simulink model "mvdc_path_feedback"  (R2018b)
settings: configuration reference "Active" (kept outside this file)
undefined symbols (not defined in the file): l_front_m, l_rear_m, P_VDC_ActivateBarriersCorrection_b, P_VDC_ActivateBetaCompensation, P_VDC_ActivateKappaDynamicFF_b, P_VDC_ActivateKappaFFFIR, P_VDC_ActivateKappaFFPT1, P_VDC_BarrierCorrectionGain_radpmpm, P_VDC_BarrierEmergency_radpm, P_VDC_BarriersCorrectionPT1_s, P_VDC_ControlMaxSpeed_mps, P_VDC_ControlMinSpeed_mps, P_VDC_CorrectionBarrierDistance_m, P_VDC_KappaFFPathFeedback_Ts, P_VDC_KappaT1_s, P_VDC_LatConvergence, P_VDC_LatDamping, P_VDC_LatKappaMaxFB_radpm, P_VDC_LatKappaMinFB_radpm, P_VDC_LongFF_PT1_s, P_VDC_MinBarrierDistance_m, P_VDC_MinSpeedGainCorrection_mps, P_VDC_NumDerivativeTFilter_s, P_VDC_UseBetaFeedback, P_VDC_UseExternalControllerParam, P_VDC_UseLongFF_PT1_b, P_VDC_UseNumDerivativePathFeedback_b, P_VDC_UseSSCDynamicsComp_b, P_VDC_UseWatchdogExternalControlParam, tS, TUMHealthStatus
libraries: simulink x10, rr_general x2
settings Model: DataDictionary=mvdc_path_feedback.sldd  Creator=wischnewski  LastModifiedBy=ge34qer

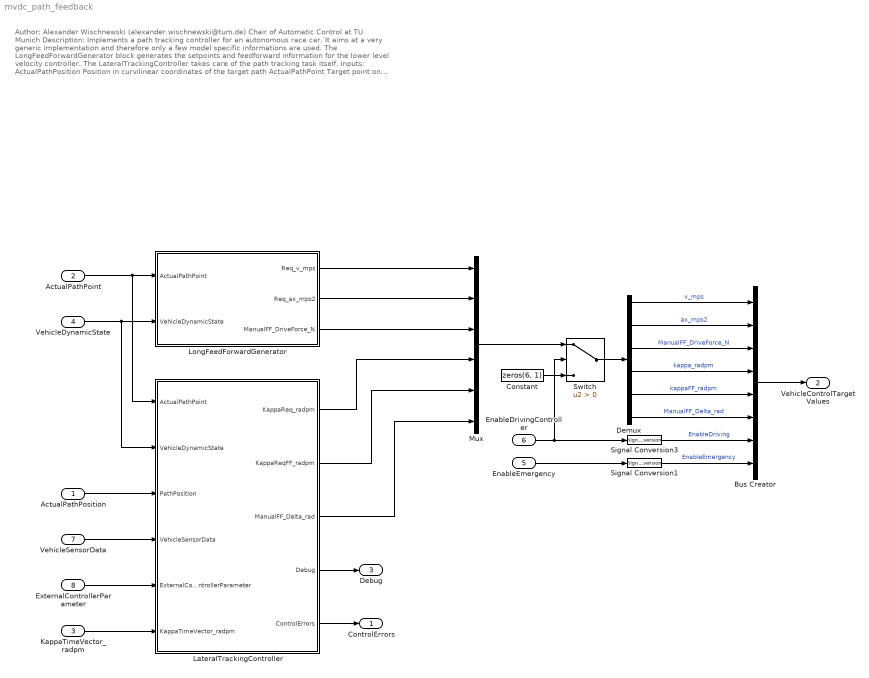
== system mvdc_path_feedback ==
  note: Author: Alexander Wischnewski (alexander.wischnewski@tum.de)
      | Chair of Automatic Control at TU Munich
      |
      | Description: Implements a path tracking controller for an autonomous race car. It aims at a very generic implementation
      | and therefore only a few model specific informations are used.
      |
      | The LongFeedForwardGenerator block generates the setpoints and feedforward information for the
      | lower level velocity controller.
      |
      | The LateralTrackingController takes care of the path tracking task itself.
      |
      | Inputs:
      | ActualPathPosition Position in curvilinear coordinates of the target path
      | ActualPathPoint Target point on the target path (found by path matching)
      | VehicleDynamicState Fused state vector of the vehicle (including position, velocity, acceleration, etc.)
      | EnableDrivingController Enable bit for controller operation
      | EnableEmergency Enable bit for emergecy control mode
      | VehicleSensorData All raw sensor data available
      | ExternalControllerParameter Interface for external modification of controller parameters (used for controller learning)
      | KappaTimeVector_radpm Vector with curvature values for a time windows of +-0.5sec
      |
      | Outputs:
      | VehicleControlTargetValues Low level controller interface of the vehicle
      | ControlErrors Outputs relevant information for controller learning
  ActualPathPosition : Inport  OutDataTypeStr=Bus: PathPos  PortDimensions=1  BusOutputAsStruct=on
  ActualPathPoint : Inport  Port=2  OutDataTypeStr=Bus: PathPoint  PortDimensions=1  BusOutputAsStruct=on
  KappaTimeVector_radpm : Inport  Port=3  PortDimensions=501  BusOutputAsStruct=on
  VehicleDynamicState : Inport  Port=4  OutDataTypeStr=Bus: VehicleDynamicState
  EnableEmergency : Inport  Port=5  OutDataTypeStr=boolean  PortDimensions=1  BusOutputAsStruct=on
  EnableDrivingController : Inport  Port=6  OutDataTypeStr=boolean  PortDimensions=1  BusOutputAsStruct=on
  VehicleSensorData : Inport  Port=7  OutDataTypeStr=Bus: VehicleSensorData  PortDimensions=1  BusOutputAsStruct=on
  ExternalControllerParameter : Inport  Port=8  OutDataTypeStr=Bus: ControllerParameter  BusOutputAsStruct=on
  Bus Creator : BusCreator  Inputs=8  OutDataTypeStr=Bus: TargetValuesVehicleDynamics
      settings: InheritFromInputs=off
  Constant : Constant  Value=zeros(6, 1)
  Demux : Demux  Outputs=6
  LateralTrackingController : Subsystem
  LongFeedForwardGenerator : Subsystem
  Mux : Mux  Inputs=6
  Signal Conversion1 : SignalConversion  OverrideOpt=off
  Signal Conversion3 : SignalConversion  OverrideOpt=off
  Switch : Switch  Criteria=u2 > Threshold
  ControlErrors : Outport  OutDataTypeStr=Bus: ControlErrors
  VehicleControlTargetValues : Outport  Port=2  OutDataTypeStr=Bus: TargetValuesVehicleDynamics
  Debug : Outport  Port=3  OutDataTypeStr=Bus: mvdc_path_feedback_debug
  wires:
  ActualPathPoint/1 -> LateralTrackingController/1(ActualPathPoint), LongFeedForwardGenerator/1(ActualPathPoint)
  ActualPathPosition/1 -> LateralTrackingController/3(PathPosition)
  VehicleDynamicState/1 -> LateralTrackingController/2(VehicleDynamicState), LongFeedForwardGenerator/2(VehicleDynamicState)
  Bus Creator/1 -> VehicleControlTargetValues/1
  Demux/5 -> Bus Creator/5  "kappaFF_radpm"
  Demux/4 -> Bus Creator/4  "kappa_radpm"
  Demux/1 -> Bus Creator/1  "v_mps"
  Demux/2 -> Bus Creator/2  "ax_mps2"
  EnableDrivingController/1 -> Switch/2, Signal Conversion3/1
  Signal Conversion3/1 -> Bus Creator/7  "EnableDriving"
  Signal Conversion1/1 -> Bus Creator/8  "EnableEmergency"
  EnableEmergency/1 -> Signal Conversion1/1
  LongFeedForwardGenerator/1(Req_v_mps) -> Mux/1
  LongFeedForwardGenerator/2(Req_ax_mps2) -> Mux/2
  LateralTrackingController/1(KappaReq_radpm) -> Mux/4
  LateralTrackingController/2(KappaReqFF_radpm) -> Mux/5
  Mux/1 -> Switch/1
  Constant/1 -> Switch/3
  Switch/1 -> Demux/1
  LateralTrackingController/4(Debug) -> Debug/1
  VehicleSensorData/1 -> LateralTrackingController/4(VehicleSensorData)
  Demux/6 -> Bus Creator/6  "ManualFF_Delta_rad"
  Demux/3 -> Bus Creator/3  "ManualFF_DriveForce_N"
  ExternalControllerParameter/1 -> LateralTrackingController/5(ExternalControllerParameter)
  KappaTimeVector_radpm/1 -> LateralTrackingController/6(KappaTimeVector_radpm)
  LongFeedForwardGenerator/3(ManualFF_DriveForce_N) -> Mux/3
  LateralTrackingController/3(ManualFF_Delta_rad) -> Mux/6
  LateralTrackingController/5(ControlErrors) -> ControlErrors/1

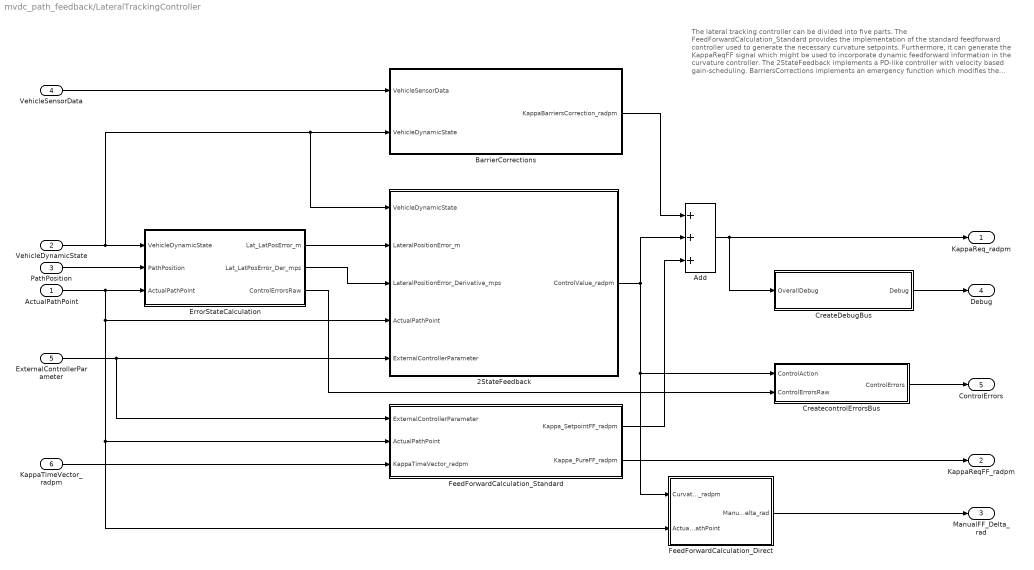
== system mvdc_path_feedback/LateralTrackingController ==
  note: The lateral tracking controller can be divided into five parts.
      |
      | The FeedForwardCalculation_Standard provides the implementation
      | of the standard feedforward controller used to generate the necessary curvature setpoints.
      | Furthermore, it can generate the KappaReqFF signal which might be used to incorporate
      | dynamic feedforward information in the curvature controller.
      |
      | The 2StateFeedback implements a PD-like controller with velocity based gain-scheduling.
      |
      | BarriersCorrections implements an emergency function which modifies the target curvature
      | signals in case barriers are near.
      |
      | ErrorStateCalculation generates the necessary control error values and its derivatives.
      |
      | Finally, FeedForwardCalculation_Direct uses a potentially available steering feedforward
      | value instead of the path curvature to generate the feedforward information. This is handed
      | directly to the lower level controller.
  ActualPathPoint : Inport  OutDataTypeStr=Bus: PathPoint
  VehicleDynamicState : Inport  Port=2  OutDataTypeStr=Bus: VehicleDynamicState
  PathPosition : Inport  Port=3
  VehicleSensorData : Inport  Port=4  OutDataTypeStr=Bus: VehicleSensorData
  ExternalControllerParameter : Inport  Port=5  BusOutputAsStruct=on
  KappaTimeVector_radpm : Inport  Port=6  PortDimensions=501  BusOutputAsStruct=on
  2StateFeedback : Subsystem
  Add : Sum  Inputs=3
  BarrierCorrections : Subsystem
  CreateDebugBus : Subsystem
  CreatecontrolErrorsBus : Subsystem
  ErrorStateCalculation : Subsystem
  FeedForwardCalculation_Direct : Subsystem
  FeedForwardCalculation_Standard : Subsystem
  KappaReq_radpm : Outport
  KappaReqFF_radpm : Outport  Port=2
  ManualFF_Delta_rad : Outport  Port=3
  Debug : Outport  Port=4
  ControlErrors : Outport  Port=5
  wires:
  Add/1 -> KappaReq_radpm/1, CreateDebugBus/1(OverallDebug)
  2StateFeedback/1(ControlValue_radpm) -> FeedForwardCalculation_Direct/1(CurvatureFeedback_radpm), CreatecontrolErrorsBus/1(ControlAction), Add/2
  FeedForwardCalculation_Standard/2(Kappa_PureFF_radpm) -> KappaReqFF_radpm/1
  VehicleDynamicState/1 -> BarrierCorrections/2(VehicleDynamicState), 2StateFeedback/1(VehicleDynamicState), ErrorStateCalculation/1(VehicleDynamicState)
  BarrierCorrections/1(KappaBarriersCorrection_radpm) -> Add/1
  ExternalControllerParameter/1 -> 2StateFeedback/5(ExternalControllerParameter), FeedForwardCalculation_Standard/1(ExternalControllerParameter)
  VehicleSensorData/1 -> BarrierCorrections/1(VehicleSensorData)
  ErrorStateCalculation/1(Lat_LatPosError_m) -> 2StateFeedback/2(LateralPositionError_m)
  PathPosition/1 -> ErrorStateCalculation/2(PathPosition)
  ErrorStateCalculation/2(Lat_LatPosError_Der_mps) -> 2StateFeedback/3(LateralPositionError_Derivative_mps)
  ActualPathPoint/1 -> FeedForwardCalculation_Direct/2(ActualPathPoint), FeedForwardCalculation_Standard/2(ActualPathPoint), 2StateFeedback/4(ActualPathPoint), ErrorStateCalculation/3(ActualPathPoint)
  FeedForwardCalculation_Standard/1(Kappa_SetpointFF_radpm) -> Add/3
  KappaTimeVector_radpm/1 -> FeedForwardCalculation_Standard/3(KappaTimeVector_radpm)
  CreateDebugBus/1(Debug) -> Debug/1
  FeedForwardCalculation_Direct/1(ManualFF_Delta_rad) -> ManualFF_Delta_rad/1
  ErrorStateCalculation/3(ControlErrorsRaw) -> CreatecontrolErrorsBus/2(ControlErrorsRaw)
  CreatecontrolErrorsBus/1(ControlErrors) -> ControlErrors/1

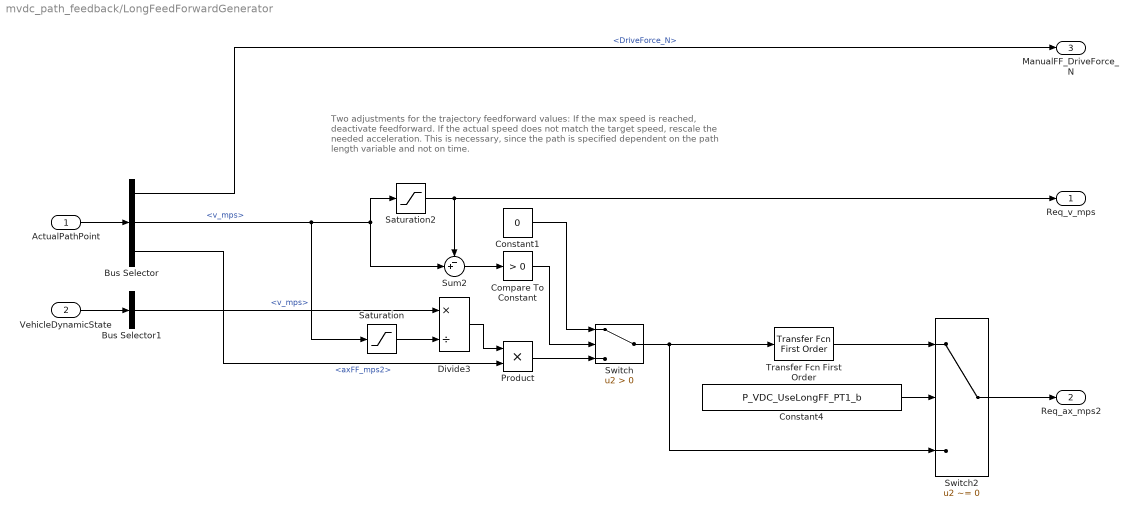
== system mvdc_path_feedback/LongFeedForwardGenerator ==
  note: Two adjustments for the trajectory feedforward values:
      | If the max speed is reached, deactivate feedforward.
      | If the actual speed does not match the target speed, rescale the needed acceleration.
      | This is necessary, since the path is specified dependent on the path length variable and
      | not on time.
  ActualPathPoint : Inport
  VehicleDynamicState : Inport  Port=2
  Bus Selector : BusSelector  OutputSignals=DriveForce_N,v_mps,axFF_mps2
  Bus Selector1 : BusSelector  OutputSignals=v_mps
  Compare To Constant : simulink/Logic and Bit Operations/Compare To Constant  relop=>  const=0  OutDataTypeStr=boolean
  Constant1 : Constant  Value=0
  Constant4 : Constant  Value=P_VDC_UseLongFF_PT1_b
  Divide3 : Product  Inputs=*/
  Product : Product
  Saturation : Saturate  UpperLimit=inf  LowerLimit=2
  Saturation2 : Saturate  UpperLimit=P_VDC_ControlMaxSpeed_mps  LowerLimit=P_VDC_ControlMinSpeed_mps
  Sum2 : Sum  Inputs=-+|
  Switch : Switch  Criteria=u2 > Threshold
  Switch2 : Switch  Criteria=u2 ~= 0
  Transfer Fcn First Order : simulink/Discrete/Transfer Fcn First Order  PoleZ=exp(-tS/P_VDC_LongFF_PT1_s)  ICPrevOutput=0.0  DoSatur=off
      settings: SourceProductName=Simulink
  Req_v_mps : Outport
  Req_ax_mps2 : Outport  Port=2
  ManualFF_DriveForce_N : Outport  Port=3
  wires:
  Constant1/1 -> Switch/1
  Sum2/1 -> Compare To Constant/1
  Compare To Constant/1 -> Switch/2
  Product/1 -> Switch/3
  Saturation/1 -> Divide3/2
  Divide3/1 -> Product/1
  Bus Selector/3 -> Product/2  "<axFF_mps2>"
  Bus Selector/2 -> Saturation/1, Saturation2/1, Sum2/2  "<v_mps>"
  Saturation2/1 -> Req_v_mps/1, Sum2/1
  Switch/1 -> Switch2/3, Transfer Fcn First Order/1
  Constant4/1 -> Switch2/2
  Transfer Fcn First Order/1 -> Switch2/1
  Switch2/1 -> Req_ax_mps2/1
  ActualPathPoint/1 -> Bus Selector/1
  VehicleDynamicState/1 -> Bus Selector1/1
  Bus Selector1/1 -> Divide3/1  "<v_mps>"
  Bus Selector/1 -> ManualFF_DriveForce_N/1  "<DriveForce_N>"

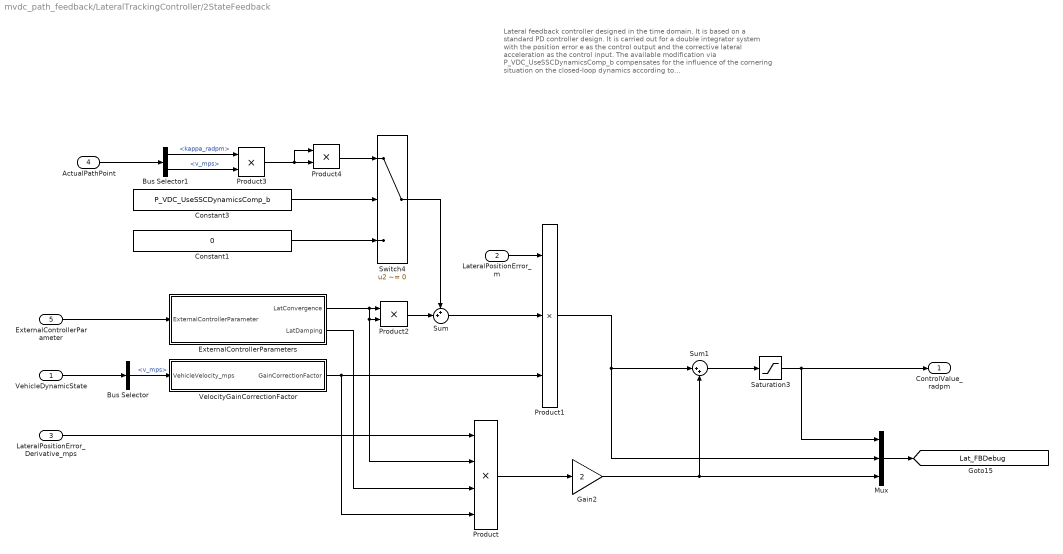
== system mvdc_path_feedback/LateralTrackingController/2StateFeedback ==
  note: Lateral feedback controller designed in the time domain. It is based on a standard PD controller design. It is carried out for a double integrator system with the position error e as the control output and the corrective lateral acceleration as the control input. The available modification via P_VDC_UseSSCDynamicsComp_b compensates for the influence of the cornering situation on the closed-loop dynamics according to
      | https://ieeexplore.ieee.org/document/6580852
      |
      | The final value is transformed to an equivalent curvature signal by using the velocity gain correction factor .
      |
      | The external controller parameters block allows to interface the controller from an other algorithm. This is used for controller learning.
  VehicleDynamicState : Inport
  LateralPositionError_m : Inport  Port=2
  LateralPositionError_Derivative_mps : Inport  Port=3
  ActualPathPoint : Inport  Port=4  OutDataTypeStr=Bus: PathPoint
  ExternalControllerParameter : Inport  Port=5  BusOutputAsStruct=on
  Bus Selector : BusSelector  OutputSignals=v_mps
  Bus Selector1 : BusSelector  OutputSignals=kappa_radpm,v_mps
  Constant1 : Constant  Value=0
  Constant3 : Constant  Value=P_VDC_UseSSCDynamicsComp_b
  ExternalControllerParameters : Subsystem
  Gain2 : Gain  Gain=2
  Mux : Mux  Inputs=3
  Product : Product  Inputs=4
  Product1 : Product  Inputs=3
  Product2 : Product
  Product3 : Product
  Product4 : Product
  Saturation3 : Saturate  UpperLimit=P_VDC_LatKappaMaxFB_radpm  LowerLimit=P_VDC_LatKappaMinFB_radpm
  Sum : Sum  Inputs=++|
  Sum1 : Sum  Inputs=|++
  Switch4 : Switch  Criteria=u2 ~= 0
  VelocityGainCorrectionFactor : Subsystem
  ControlValue_radpm : Outport
  tag scope: Lat_FBDebug=global
  wires:
  LateralPositionError_m/1 -> Product1/1
  Product/1 -> Gain2/1
  ExternalControllerParameters/2(LatDamping) -> Product/3
  ExternalControllerParameters/1(LatConvergence) -> Product2/2, Product/2, Product2/1
  VelocityGainCorrectionFactor/1(GainCorrectionFactor) -> Product1/3, Product/4
  Sum1/1 -> Saturation3/1
  ExternalControllerParameter/1 -> ExternalControllerParameters/1(ExternalControllerParameter)
  VehicleDynamicState/1 -> Bus Selector/1
  Bus Selector/1 -> VelocityGainCorrectionFactor/1(VehicleVelocity_mps)  "<v_mps>"
  Saturation3/1 -> Mux/1, ControlValue_radpm/1
  Product1/1 -> Mux/2, Sum1/1
  Gain2/1 -> Mux/3, Sum1/2
  Mux/1 -> [Lat_FBDebug]
  Product2/1 -> Sum/2
  Sum/1 -> Product1/2
  Product3/1 -> Product4/1, Product4/2
  ActualPathPoint/1 -> Bus Selector1/1
  Bus Selector1/1 -> Product3/1  "<kappa_radpm>"
  Bus Selector1/2 -> Product3/2  "<v_mps>"
  Constant3/1 -> Switch4/2
  Product4/1 -> Switch4/1
  Switch4/1 -> Sum/1
  Constant1/1 -> Switch4/3
  LateralPositionError_Derivative_mps/1 -> Product/1

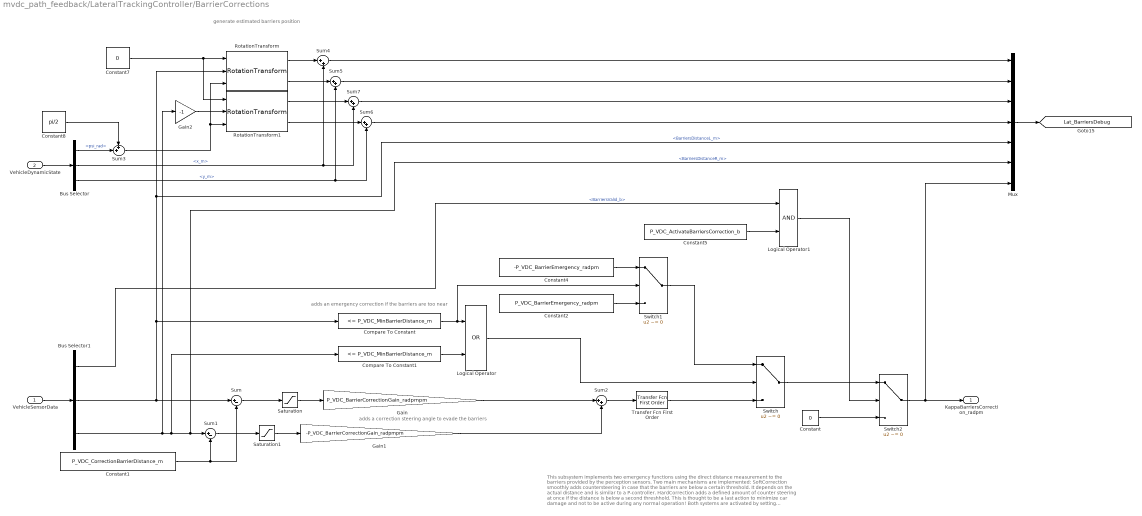
== system mvdc_path_feedback/LateralTrackingController/BarrierCorrections ==
  note: This subsystem implements two emergency functions using the direct distance measurement
      | to the barriers provided by the perception sensors.
      |
      | Two main mechanisms are implemented:
      | SoftCorrection smoothly adds countersteering in case that the barriers are below a certain threshold. It depends
      | on the actual distance and is similar to a P-controller.
      | HardCorrection adds a defined amount of counter steering at once if the distance is below a second threshhold.
      | This is thought to be a last action to minimize car damage and not to be active during any normal operation!
      |
      | Both systems are activated by setting P_VDC_ActivateBarriersCorrection_b to true.
  note: generate estimated barriers position
  note: adds an emergency correction if the barriers are too near
  note: adds a correction steering angle to evade the barriers
  VehicleSensorData : Inport
  VehicleDynamicState : Inport  Port=2
  Bus Selector : BusSelector  OutputSignals=Pos.psi_rad,Pos.x_m,Pos.y_m
  Bus Selector1 : BusSelector  OutputSignals=BarriersValid_b,BarriersDistanceL_m,BarriersDistanceR_m
  Compare To Constant : simulink/Logic and Bit Operations/Compare To Constant  relop=<=  const=P_VDC_MinBarrierDistance_m  OutDataTypeStr=boolean
  Compare To Constant1 : simulink/Logic and Bit Operations/Compare To Constant  relop=<=  const=P_VDC_MinBarrierDistance_m  OutDataTypeStr=boolean
  Constant : Constant  Value=0
  Constant1 : Constant  Value=P_VDC_CorrectionBarrierDistance_m
  Constant2 : Constant  Value=P_VDC_BarrierEmergency_radpm
  Constant4 : Constant  Value=-P_VDC_BarrierEmergency_radpm
  Constant5 : Constant  Value=P_VDC_ActivateBarriersCorrection_b
  Constant7 : Constant  Value=0
  Constant8 : Constant  Value=pi/2
  Gain : Gain  Gain=P_VDC_BarrierCorrectionGain_radpmpm
  Gain1 : Gain  Gain=-P_VDC_BarrierCorrectionGain_radpmpm
  Gain2 : Gain  Gain=-1
  Logical Operator : Logic  Operator=OR  AllPortsSameDT=off  OutDataTypeStr=boolean
  Logical Operator1 : Logic  AllPortsSameDT=off  OutDataTypeStr=boolean
  Mux : Mux  Inputs=7
  RotationTransform : rr_general/RotationTransform  SystemSampleTime=-1
  RotationTransform1 : rr_general/RotationTransform  SystemSampleTime=-1
  Saturation : Saturate  UpperLimit=0  LowerLimit=-(P_VDC_CorrectionBarrierDistance_m-P_VDC_MinBarrierDistance_m)
  Saturation1 : Saturate  UpperLimit=0  LowerLimit=-(P_VDC_CorrectionBarrierDistance_m-P_VDC_MinBarrierDistance_m)
  Sum : Sum  Inputs=|+-
  Sum1 : Sum  Inputs=|+-
  Sum{2,4..7} (5 alike) : Sum  Inputs=|++
  Sum3 : Sum  Inputs=++|
  Switch : Switch  Criteria=u2 ~= 0
  Switch1 : Switch  Criteria=u2 ~= 0
  Switch2 : Switch  Criteria=u2 ~= 0
  Transfer Fcn First Order : simulink/Discrete/Transfer Fcn First Order  PoleZ=exp(-tS/P_VDC_BarriersCorrectionPT1_s)  ICPrevOutput=0.0  DoSatur=off
      settings: SourceProductName=Simulink
  KappaBarriersCorrection_radpm : Outport
  tag scope: Lat_BarriersDebug=global
  wires:
  Bus Selector1/3 -> Gain2/1, Compare To Constant1/1, Mux/6, Sum1/1  "<BarriersDistanceR_m>"
  Constant1/1 -> Sum/2, Sum1/2
  Sum/1 -> Saturation/1
  Sum1/1 -> Saturation1/1
  Saturation/1 -> Gain/1
  Saturation1/1 -> Gain1/1
  Gain/1 -> Sum2/1
  Gain1/1 -> Sum2/2
  Sum2/1 -> Transfer Fcn First Order/1
  Compare To Constant1/1 -> Logical Operator/2
  Compare To Constant/1 -> Switch1/2, Logical Operator/1
  Transfer Fcn First Order/1 -> Switch/3
  Logical Operator/1 -> Switch/2
  Switch1/1 -> Switch/1
  Constant2/1 -> Switch1/3
  Constant4/1 -> Switch1/1
  Switch/1 -> Switch2/1
  Switch2/1 -> Mux/7, KappaBarriersCorrection_radpm/1
  Constant/1 -> Switch2/3
  Logical Operator1/1 -> Switch2/2
  Gain2/1 -> RotationTransform1/2
  Constant7/1 -> RotationTransform1/1, RotationTransform/1
  VehicleDynamicState/1 -> Bus Selector/1
  Sum3/1 -> RotationTransform/3, RotationTransform1/3
  Bus Selector/1 -> Sum3/2  "<psi_rad>"
  Constant8/1 -> Sum3/1
  RotationTransform/1 -> Sum4/1
  Bus Selector/2 -> Sum7/2, Sum4/2  "<x_m>"
  RotationTransform/2 -> Sum5/1
  Bus Selector/3 -> Sum6/2, Sum5/2  "<y_m>"
  RotationTransform1/2 -> Sum6/1
  RotationTransform1/1 -> Sum7/1
  Sum6/1 -> Mux/4
  Sum7/1 -> Mux/3
  Sum5/1 -> Mux/2
  Sum4/1 -> Mux/1
  Bus Selector1/2 -> Mux/5, RotationTransform/2, Compare To Constant/1, Sum/1  "<BarriersDistanceL_m>"
  Constant5/1 -> Logical Operator1/2
  Bus Selector1/1 -> Logical Operator1/1  "<BarriersValid_b>"
  VehicleSensorData/1 -> Bus Selector1/1
  Mux/1 -> [Lat_BarriersDebug]

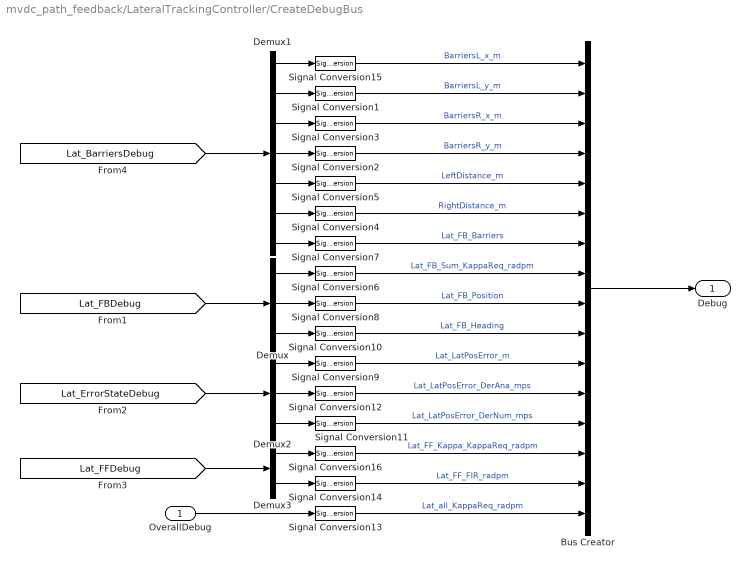
== system mvdc_path_feedback/LateralTrackingController/CreateDebugBus ==
  OverallDebug : Inport
  Bus Creator : BusCreator  Inputs=16
  Demux : Demux  Outputs=3
  Demux1 : Demux  Outputs=7
  Demux2 : Demux  Outputs=3
  Demux3 : Demux  Outputs=2
  Signal Conversion{1..16} (16 alike) : SignalConversion  OverrideOpt=off
  Debug : Outport
  wires:
  [Lat_FBDebug] -> Demux/1
  Demux3/2 -> Signal Conversion14/1
  Demux2/1 -> Signal Conversion9/1
  Demux1/3 -> Signal Conversion3/1
  Demux1/7 -> Signal Conversion7/1
  OverallDebug/1 -> Signal Conversion13/1
  Demux1/2 -> Signal Conversion1/1
  Demux1/1 -> Signal Conversion15/1
  Demux/2 -> Signal Conversion8/1
  Demux2/2 -> Signal Conversion12/1
  Demux2/3 -> Signal Conversion11/1
  Demux3/1 -> Signal Conversion16/1
  Demux1/6 -> Signal Conversion4/1
  [Lat_FFDebug] -> Demux3/1
  Bus Creator/1 -> Debug/1
  Demux1/4 -> Signal Conversion2/1
  Demux1/5 -> Signal Conversion5/1
  Demux/1 -> Signal Conversion6/1
  Demux/3 -> Signal Conversion10/1
  [Lat_ErrorStateDebug] -> Demux2/1
  [Lat_BarriersDebug] -> Demux1/1
  Signal Conversion15/1 -> Bus Creator/1  "BarriersL_x_m"
  Signal Conversion1/1 -> Bus Creator/2  "BarriersL_y_m"
  Signal Conversion2/1 -> Bus Creator/4  "BarriersR_y_m"
  Signal Conversion3/1 -> Bus Creator/3  "BarriersR_x_m"
  Signal Conversion4/1 -> Bus Creator/6  "RightDistance_m"
  Signal Conversion7/1 -> Bus Creator/7  "Lat_FB_Barriers"
  Signal Conversion5/1 -> Bus Creator/5  "LeftDistance_m"
  Signal Conversion6/1 -> Bus Creator/8  "Lat_FB_Sum_KappaReq_radpm"
  Signal Conversion8/1 -> Bus Creator/9  "Lat_FB_Position"
  Signal Conversion11/1 -> Bus Creator/13  "Lat_LatPosError_DerNum_mps"
  Signal Conversion9/1 -> Bus Creator/11  "Lat_LatPosError_m"
  Signal Conversion10/1 -> Bus Creator/10  "Lat_FB_Heading"
  Signal Conversion12/1 -> Bus Creator/12  "Lat_LatPosError_DerAna_mps"
  Signal Conversion13/1 -> Bus Creator/16  "Lat_all_KappaReq_radpm"
  Signal Conversion14/1 -> Bus Creator/15  "Lat_FF_FIR_radpm"
  Signal Conversion16/1 -> Bus Creator/14  "Lat_FF_Kappa_KappaReq_radpm"

== system mvdc_path_feedback/LateralTrackingController/CreatecontrolErrorsBus ==
  ControlAction : Inport
  ControlErrorsRaw : Inport  Port=2
  Bus Creator : BusCreator  Inputs=4
  Demux : Demux  Outputs=3
  ControlErrors : Outport
  wires:
  Bus Creator/1 -> ControlErrors/1
  Demux/1 -> Bus Creator/1  "e_LateralDeviation_m"
  Demux/2 -> Bus Creator/2  "de_LateralDeviationDer_mps"
  Demux/3 -> Bus Creator/3  "ePsi_HeadingDeviation_rad"
  ControlErrorsRaw/1 -> Demux/1
  ControlAction/1 -> Bus Creator/4  "u_ControlInput_radpm"

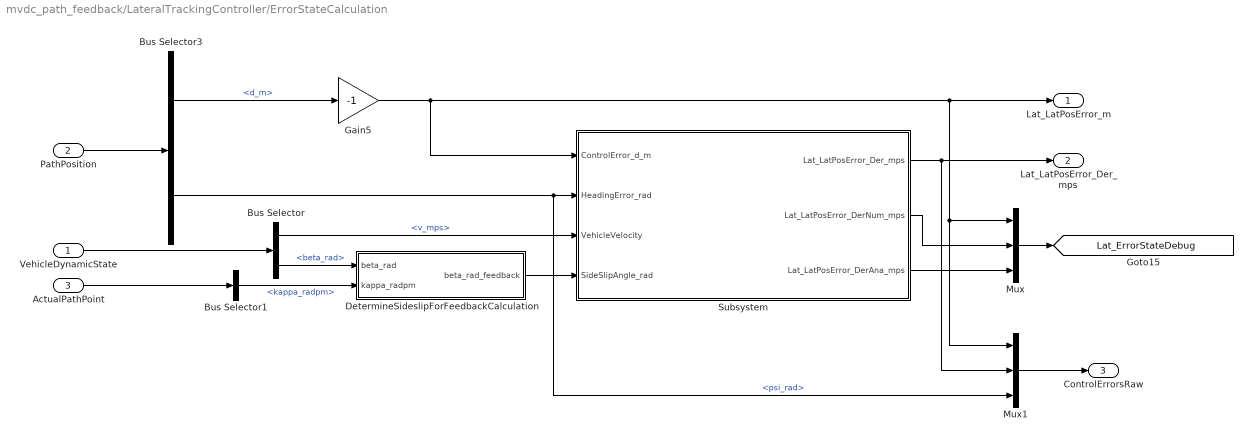
== system mvdc_path_feedback/LateralTrackingController/ErrorStateCalculation ==
  VehicleDynamicState : Inport
  PathPosition : Inport  Port=2
  ActualPathPoint : Inport  Port=3
  Bus Selector : BusSelector  OutputSignals=v_mps,beta_rad
  Bus Selector1 : BusSelector  OutputSignals=kappa_radpm
  Bus Selector3 : BusSelector  OutputSignals=d_m,psi_rad
  DetermineSideslipForFeedbackCalculation : Subsystem
  Gain5 : Gain  Gain=-1
  Mux : Mux  Inputs=3
  Mux1 : Mux  Inputs=3
  Subsystem : Subsystem
  Lat_LatPosError_m : Outport
  Lat_LatPosError_Der_mps : Outport  Port=2
  ControlErrorsRaw : Outport  Port=3
  tag scope: Lat_ErrorStateDebug=global
  wires:
  Gain5/1 -> Mux1/1, Mux/1, Lat_LatPosError_m/1, Subsystem/1(ControlError_d_m)
  VehicleDynamicState/1 -> Bus Selector/1
  Bus Selector3/1 -> Gain5/1  "<d_m>"
  PathPosition/1 -> Bus Selector3/1
  ActualPathPoint/1 -> Bus Selector1/1
  Bus Selector/2 -> DetermineSideslipForFeedbackCalculation/1(beta_rad)  "<beta_rad>"
  Bus Selector1/1 -> DetermineSideslipForFeedbackCalculation/2(kappa_radpm)  "<kappa_radpm>"
  Bus Selector3/2 -> Mux1/3, Subsystem/2(HeadingError_rad)  "<psi_rad>"
  DetermineSideslipForFeedbackCalculation/1(beta_rad_feedback) -> Subsystem/4(SideSlipAngle_rad)
  Subsystem/1(Lat_LatPosError_Der_mps) -> Mux1/2, Lat_LatPosError_Der_mps/1
  Bus Selector/1 -> Subsystem/3(VehicleVelocity)  "<v_mps>"
  Subsystem/2(Lat_LatPosError_DerNum_mps) -> Mux/2
  Subsystem/3(Lat_LatPosError_DerAna_mps) -> Mux/3
  Mux/1 -> [Lat_ErrorStateDebug]
  Mux1/1 -> ControlErrorsRaw/1

== system mvdc_path_feedback/LateralTrackingController/FeedForwardCalculation_Direct ==
  CurvatureFeedback_radpm : Inport  BusOutputAsStruct=on
  ActualPathPoint : Inport  Port=2
  Bus Selector : BusSelector  OutputSignals=Delta_rad
  Sum : Sum  Inputs=|++
  ManualFF_Delta_rad : Outport
  wires:
  CurvatureFeedback_radpm/1 -> Sum/1
  ActualPathPoint/1 -> Bus Selector/1
  Bus Selector/1 -> Sum/2  "<Delta_rad>"
  Sum/1 -> ManualFF_Delta_rad/1

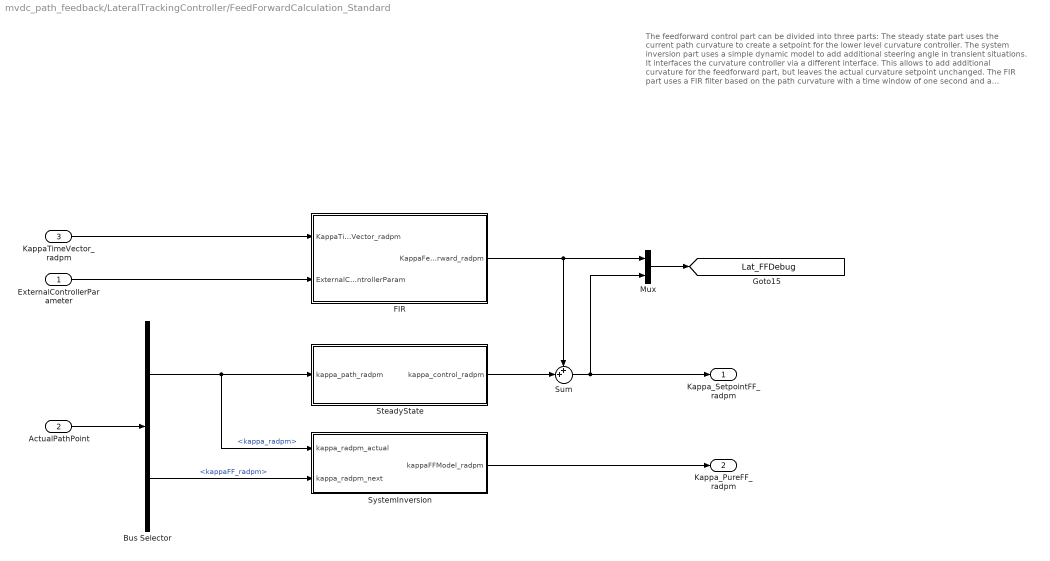
== system mvdc_path_feedback/LateralTrackingController/FeedForwardCalculation_Standard ==
  note: The feedforward control part can be divided into three parts:
      |
      | The steady state part uses the current path curvature to create a setpoint
      | for the lower level curvature controller.
      |
      | The system inversion part uses a simple dynamic model to add additional steering
      | angle in transient situations. It interfaces the curvature controller via a different interface.
      | This allows to add additional curvature for the feedforward part, but leaves the actual
      | curvature setpoint unchanged.
      |
      | The FIR part uses a FIR filter based on the path curvature with a time window of one second
      | and a foresight of half a second. Its coefficients can be set externally. This is used for
      | controller learning and should be deactivated in most cases.
  ExternalControllerParameter : Inport  BusOutputAsStruct=on
  ActualPathPoint : Inport  Port=2
  KappaTimeVector_radpm : Inport  Port=3  PortDimensions=501  BusOutputAsStruct=on
  Bus Selector : BusSelector  OutputSignals=kappa_radpm,kappaFF_radpm
  FIR : Subsystem
  Mux : Mux  Inputs=2
  SteadyState : Subsystem
  Sum : Sum  Inputs=++|
  SystemInversion : Subsystem
  Kappa_SetpointFF_radpm : Outport
  Kappa_PureFF_radpm : Outport  Port=2
  tag scope: Lat_FFDebug=global
  wires:
  SystemInversion/1(kappaFFModel_radpm) -> Kappa_PureFF_radpm/1
  Bus Selector/1 -> SystemInversion/1(kappa_radpm_actual), SteadyState/1(kappa_path_radpm)  "<kappa_radpm>"
  Bus Selector/2 -> SystemInversion/2(kappa_radpm_next)  "<kappaFF_radpm>"
  KappaTimeVector_radpm/1 -> FIR/1(KappaTimeVector_radpm)
  ExternalControllerParameter/1 -> FIR/2(ExternalControllerParam)
  ActualPathPoint/1 -> Bus Selector/1
  Sum/1 -> Mux/2, Kappa_SetpointFF_radpm/1
  FIR/1(KappaFeedForward_radpm) -> Mux/1, Sum/1
  SteadyState/1(kappa_control_radpm) -> Sum/2
  Mux/1 -> [Lat_FFDebug]

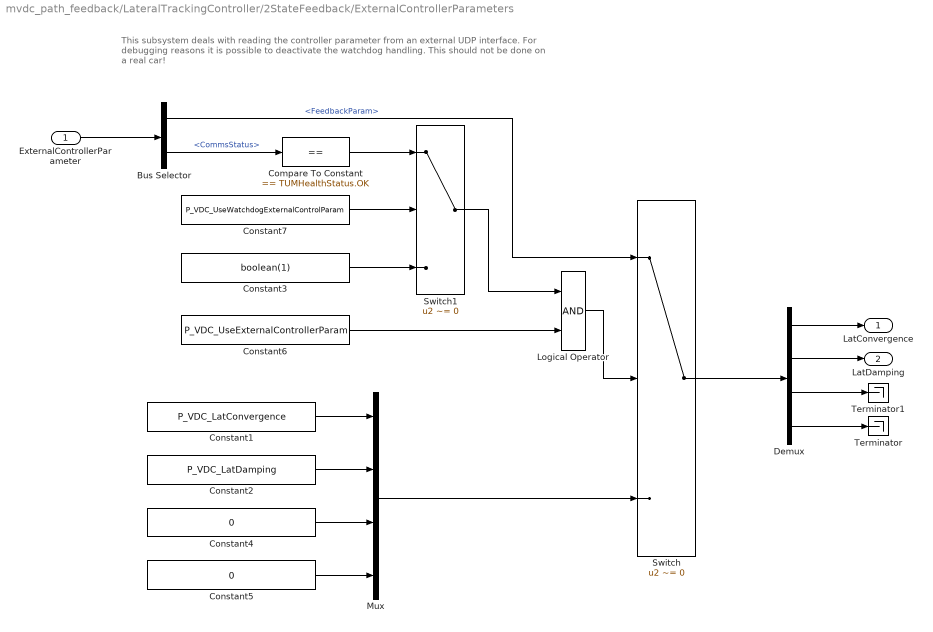
== system mvdc_path_feedback/LateralTrackingController/2StateFeedback/ExternalControllerParameters ==
  note: This subsystem deals with reading the controller parameter from an external UDP interface.
      | For debugging reasons it is possible to deactivate the watchdog handling. This should not
      | be done on a real car!
  ExternalControllerParameter : Inport
  Bus Selector : BusSelector  OutputSignals=FeedbackParam,CommsStatus
  Compare To Constant : simulink/Logic and Bit Operations/Compare To Constant  relop===  const=TUMHealthStatus.OK  OutDataTypeStr=boolean
  Constant1 : Constant  Value=P_VDC_LatConvergence
  Constant2 : Constant  Value=P_VDC_LatDamping
  Constant3 : Constant  Value=boolean(1)
  Constant4 : Constant  Value=0
  Constant5 : Constant  Value=0
  Constant6 : Constant  Value=P_VDC_UseExternalControllerParam
  Constant7 : Constant  Value=P_VDC_UseWatchdogExternalControlParam
  Demux : Demux
  Logical Operator : Logic  AllPortsSameDT=off  OutDataTypeStr=boolean
  Mux : Mux
  Switch : Switch  Criteria=u2 ~= 0
  Switch1 : Switch  Criteria=u2 ~= 0
  Terminator : Terminator
  Terminator1 : Terminator
  LatConvergence : Outport
  LatDamping : Outport  Port=2
  wires:
  Constant2/1 -> Mux/2
  Mux/1 -> Switch/3
  Constant1/1 -> Mux/1
  Constant4/1 -> Mux/3
  Constant5/1 -> Mux/4
  Switch/1 -> Demux/1
  Demux/3 -> Terminator1/1
  Demux/4 -> Terminator/1
  Demux/1 -> LatConvergence/1
  Demux/2 -> LatDamping/1
  ExternalControllerParameter/1 -> Bus Selector/1
  Bus Selector/1 -> Switch/1  "<FeedbackParam>"
  Constant6/1 -> Logical Operator/2
  Logical Operator/1 -> Switch/2
  Bus Selector/2 -> Compare To Constant/1  "<CommsStatus>"
  Compare To Constant/1 -> Switch1/1
  Switch1/1 -> Logical Operator/1
  Constant3/1 -> Switch1/3
  Constant7/1 -> Switch1/2

== system mvdc_path_feedback/LateralTrackingController/2StateFeedback/VelocityGainCorrectionFactor ==
  note: The velocity gain correction factor is calculated such that the corrective acceleration
      | from the controller is mapped to an equivalent curvature request. For small velocities
      | a minimum value is used for calculation. This leads to less control effort at low speeds and
      | ensures a smooth operation of the control system. Otherwise the controller gains would
      | tend to infinity for small speeds.
  VehicleVelocity_mps : Inport
  Constant : Constant
  Constant3 : Constant  Value=P_VDC_MinSpeedGainCorrection_mps
  Divide : Product  Inputs=*/
  MinMax : MinMax  Function=max  Inputs=2
  Product : Product
  GainCorrectionFactor : Outport
  wires:
  VehicleVelocity_mps/1 -> MinMax/1
  MinMax/1 -> Divide/2
  Constant3/1 -> MinMax/2
  Constant/1 -> Divide/1
  Divide/1 -> Product/2, Product/1
  Product/1 -> GainCorrectionFactor/1

== system mvdc_path_feedback/LateralTrackingController/ErrorStateCalculation/DetermineSideslipForFeedbackCalculation ==
  note: Determines which side slip angle is used for calculation of the control
      | error derivative. Two options are available:
      |
      | Top : Use measured/estimated side slip angle. This might lead to oscillations
      | in case of noisy values. Use only with good quality side slip angle estimates.
      |
      | Bottom : Calculates the neutral steer steering angle value for the current target
      | curvature of the path. Afterwards, the chassis slip angle at the centre of gravity
      | is calculated based on a no slip assumption for the tires, this is true for small velocities.
      | This option is less sensitive to measurement quality, however the no tire slip assumption
      | is clearly false for racing purposes. This could lead to steady-state control error.
  beta_rad : Inport
  kappa_radpm : Inport  Port=2
  Constant2 : Constant  Value=P_VDC_UseBetaFeedback
  Gain1 : Gain  Gain=l_front_m+l_rear_m
  Gain2 : Gain  Gain=l_rear_m/(l_front_m+l_rear_m)
  Switch3 : Switch  Criteria=u2 > Threshold
  beta_rad_feedback : Outport
  wires:
  beta_rad/1 -> Switch3/1
  Gain2/1 -> Switch3/3
  Constant2/1 -> Switch3/2
  Switch3/1 -> beta_rad_feedback/1
  kappa_radpm/1 -> Gain1/1
  Gain1/1 -> Gain2/1

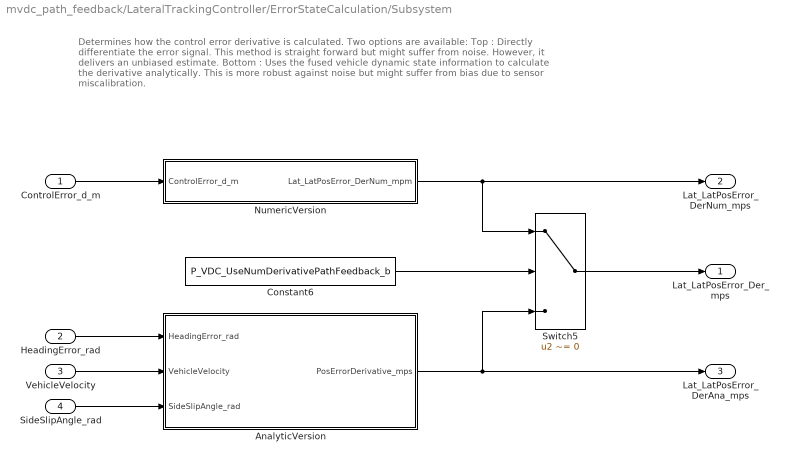
== system mvdc_path_feedback/LateralTrackingController/ErrorStateCalculation/Subsystem ==
  note: Determines how the control error derivative is calculated. Two options are available:
      |
      | Top : Directly differentiate the error signal. This method is straight forward but might suffer from
      | noise. However, it delivers an unbiased estimate.
      |
      | Bottom : Uses the fused vehicle dynamic state information to calculate the derivative analytically.
      | This is more robust against noise but might suffer from bias due to sensor miscalibration.
  ControlError_d_m : Inport
  HeadingError_rad : Inport  Port=2
  VehicleVelocity : Inport  Port=3
  SideSlipAngle_rad : Inport  Port=4
  AnalyticVersion : Subsystem
  Constant6 : Constant  Value=P_VDC_UseNumDerivativePathFeedback_b
  NumericVersion : Subsystem
  Switch5 : Switch  Criteria=u2 ~= 0
  Lat_LatPosError_Der_mps : Outport
  Lat_LatPosError_DerNum_mps : Outport  Port=2
  Lat_LatPosError_DerAna_mps : Outport  Port=3
  wires:
  HeadingError_rad/1 -> AnalyticVersion/1(HeadingError_rad)
  NumericVersion/1(Lat_LatPosError_DerNum_mpm) -> Lat_LatPosError_DerNum_mps/1, Switch5/1
  AnalyticVersion/1(PosErrorDerivative_mps) -> Switch5/3, Lat_LatPosError_DerAna_mps/1
  Switch5/1 -> Lat_LatPosError_Der_mps/1
  Constant6/1 -> Switch5/2
  ControlError_d_m/1 -> NumericVersion/1(ControlError_d_m)
  VehicleVelocity/1 -> AnalyticVersion/2(VehicleVelocity)
  SideSlipAngle_rad/1 -> AnalyticVersion/3(SideSlipAngle_rad)

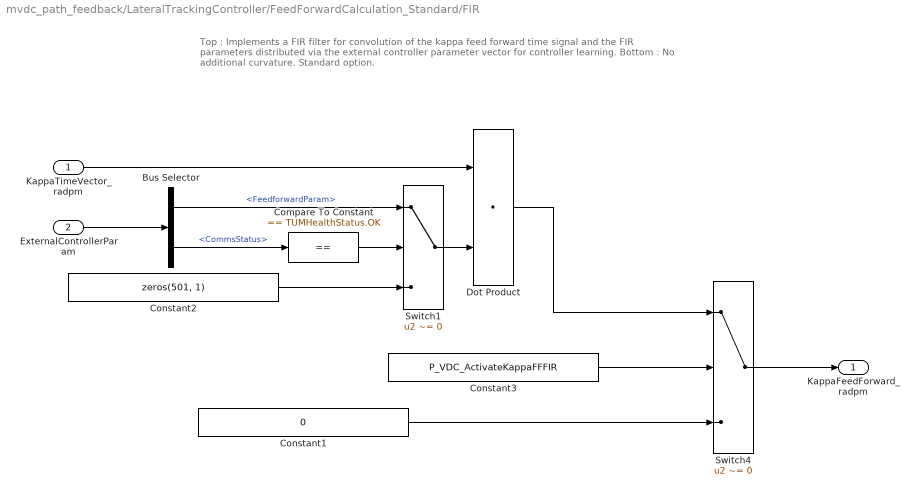
== system mvdc_path_feedback/LateralTrackingController/FeedForwardCalculation_Standard/FIR ==
  note: Top : Implements a FIR filter for convolution of the kappa feed forward time signal
      | and the FIR parameters distributed via the external controller parameter vector for controller learning.
      |
      | Bottom : No additional curvature. Standard option.
  KappaTimeVector_radpm : Inport
  ExternalControllerParam : Inport  Port=2
  Bus Selector : BusSelector  OutputSignals=FeedforwardParam,CommsStatus
  Compare To Constant : simulink/Logic and Bit Operations/Compare To Constant  relop===  const=TUMHealthStatus.OK  OutDataTypeStr=boolean
  Constant1 : Constant  Value=0
  Constant2 : Constant  Value=zeros(501, 1)
  Constant3 : Constant  Value=P_VDC_ActivateKappaFFFIR
  Dot Product : DotProduct  InputSameDT=on  OutDataTypeStr=Inherit: Inherit via internal rule
  Switch1 : Switch  Criteria=u2 ~= 0
  Switch4 : Switch  Criteria=u2 ~= 0
  KappaFeedForward_radpm : Outport
  wires:
  KappaTimeVector_radpm/1 -> Dot Product/1
  ExternalControllerParam/1 -> Bus Selector/1
  Constant3/1 -> Switch4/2
  Switch4/1 -> KappaFeedForward_radpm/1
  Dot Product/1 -> Switch4/1
  Constant1/1 -> Switch4/3
  Bus Selector/1 -> Switch1/1  "<FeedforwardParam>"
  Switch1/1 -> Dot Product/2
  Bus Selector/2 -> Compare To Constant/1  "<CommsStatus>"
  Constant2/1 -> Switch1/3
  Compare To Constant/1 -> Switch1/2

== system mvdc_path_feedback/LateralTrackingController/FeedForwardCalculation_Standard/SteadyState ==
  note: This subsystem generates the curvature which is used for setpoint generation from
      | the path curvature. Two options are available:
      |
      | Top : Apply a low pass to the actual path curvature. Might be helpful if path curvature
      | information is noisy, however its not recommended to use this. Only as a backup!
      |
      | Bottom : Direct usage of path curvature as feedforward information. Standard option.
  kappa_path_radpm : Inport
  Constant3 : Constant  Value=P_VDC_ActivateKappaFFPT1
  Switch4 : Switch  Criteria=u2 ~= 0
  Transfer Fcn First Order : simulink/Discrete/Transfer Fcn First Order  PoleZ=exp(-tS/P_VDC_KappaT1_s)  ICPrevOutput=0.0  DoSatur=off
      settings: SourceProductName=Simulink
  kappa_control_radpm : Outport
  wires:
  Transfer Fcn First Order/1 -> Switch4/1
  kappa_path_radpm/1 -> Transfer Fcn First Order/1, Switch4/3
  Switch4/1 -> kappa_control_radpm/1
  Constant3/1 -> Switch4/2

== system mvdc_path_feedback/LateralTrackingController/FeedForwardCalculation_Standard/SystemInversion ==
  note: Top : Apply an inverted first-order low pass to generate additional
      | feedforward action in transient situations. Only recommend for non-agile vehicles with high yaw inertia.
      |
      | Bottom : No additional curvature. Standard option, usually sufficient and more robust.
  kappa_radpm_actual : Inport
  kappa_radpm_next : Inport  Port=2
  Constant : Constant  Value=P_VDC_ActivateKappaDynamicFF_b
  Constant1 : Constant  Value=0
  Gain : Gain  Gain=exp(-tS/P_VDC_KappaFFPathFeedback_Ts)
  Gain1 : Gain  Gain=1/(1-exp(-tS/P_VDC_KappaFFPathFeedback_Ts))
  Sum1 : Sum  Inputs=|+-
  Sum2 : Sum  Inputs=|+-
  Switch : Switch  Criteria=u2 > Threshold
  kappaFFModel_radpm : Outport
  wires:
  Sum2/1 -> Gain1/1
  kappa_radpm_next/1 -> Sum2/1
  kappa_radpm_actual/1 -> Sum1/2, Gain/1
  Gain/1 -> Sum2/2
  Gain1/1 -> Sum1/1
  Switch/1 -> kappaFFModel_radpm/1
  Sum1/1 -> Switch/1
  Constant/1 -> Switch/2
  Constant1/1 -> Switch/3

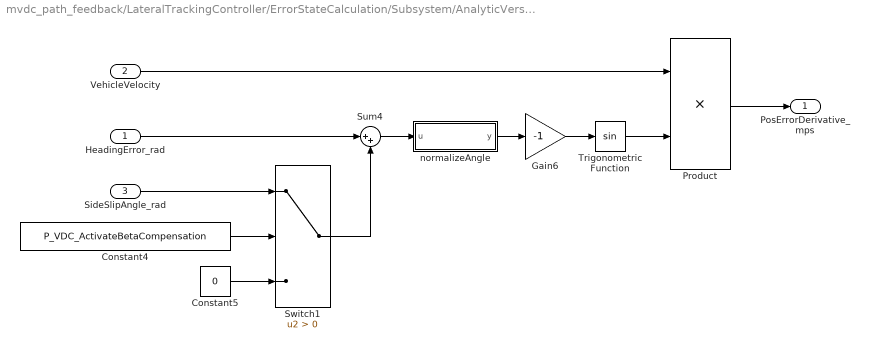
== system mvdc_path_feedback/LateralTrackingController/ErrorStateCalculation/Subsystem/AnalyticVersion ==
  HeadingError_rad : Inport
  VehicleVelocity : Inport  Port=2
  SideSlipAngle_rad : Inport  Port=3
  Constant4 : Constant  Value=P_VDC_ActivateBetaCompensation
  Constant5 : Constant  Value=0
  Gain6 : Gain  Gain=-1
  Product : Product
  Sum4 : Sum  Inputs=|++
  Switch1 : Switch  Criteria=u2 > Threshold
  Trigonometric Function : Trigonometry
  normalizeAngle : MATLAB Function  TreatAsAtomicUnit=on
  PosErrorDerivative_mps : Outport
  wires:
  VehicleVelocity/1 -> Product/1
  normalizeAngle/1(y) -> Gain6/1
  Trigonometric Function/1 -> Product/2
  Switch1/1 -> Sum4/2
  Constant4/1 -> Switch1/2
  Gain6/1 -> Trigonometric Function/1
  Constant5/1 -> Switch1/3
  Sum4/1 -> normalizeAngle/1(u)
  Product/1 -> PosErrorDerivative_mps/1
  HeadingError_rad/1 -> Sum4/1
  SideSlipAngle_rad/1 -> Switch1/1

== system mvdc_path_feedback/LateralTrackingController/ErrorStateCalculation/Subsystem/NumericVersion ==
  ControlError_d_m : Inport
  Discrete Derivative : simulink/Discrete/Discrete Derivative  gainval=1.0  ICPrevScaledInput=0.0  OutMin=[]  OutMax=[]  OutDataType=fixdt(1, 16)  OutScaling=2^-10  DoSatur=off
  Transfer Fcn First Order : simulink/Discrete/Transfer Fcn First Order  PoleZ=exp(-tS/P_VDC_NumDerivativeTFilter_s)  ICPrevOutput=0.0  DoSatur=off
      settings: SourceProductName=Simulink
  Lat_LatPosError_DerNum_mpm : Outport
  wires:
  ControlError_d_m/1 -> Discrete Derivative/1
  Transfer Fcn First Order/1 -> Lat_LatPosError_DerNum_mpm/1
  Discrete Derivative/1 -> Transfer Fcn First Order/1

== matlab function mvdc_path_feedback/LateralTrackingController/ErrorStateCalculation/Subsystem/AnalyticVersion/normalizeAngle ==
  data: u input; y output
function y = fcn(u)

y = normalizeAngle(u);
